simulink model "Bergman_Model_Non_Linear"  (R2026a)
settings: Solver=ode45  StopTime=1440
libraries: mpclib x1
settings Model: Creator=ADMIN
settings SimscapeCC: SimscapeNominalValues="[{\"value\":\"1\",\"unit\":\"A\"},{\"value\":\"1\",\"unit\":\"bar\"},{\"value\":\"1\",\"unit\":\"cm^2\"},{\"value\":\"1\",\"unit\":\"cm^3/s\"},{\"value\":\"1\",\"unit\":\"kJ/kg\"},{\"value\":\"1\",\"unit\":\"kW\"},{\"value\":\"1\",\"unit\":\"l\"},{\"value\":\"1\",\"unit\":\"N\"},{\"value\":\"1\",\"unit\":\"N*m\"},{\"value\":\"1\",\"unit\":\"V\"}]"  SimscapeLogType=none  SimscapeLogDataHistory=5000.0

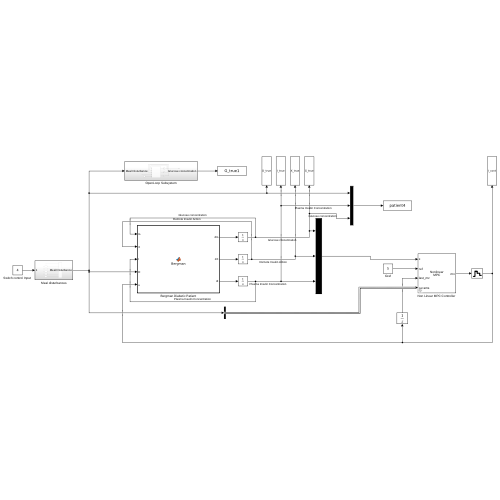
[thumbnail: Simulink's stored preview of the top-level diagram]
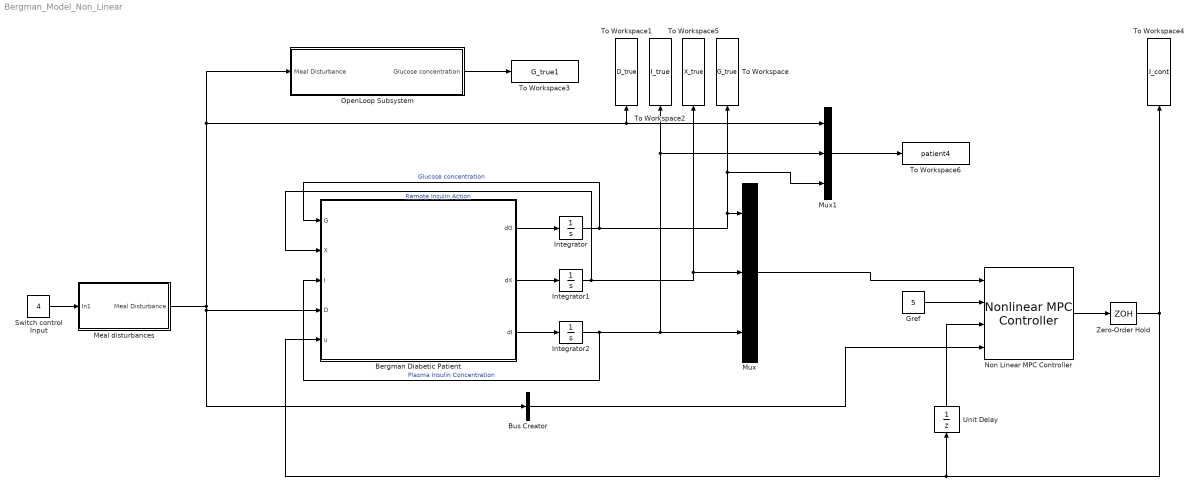
== system Bergman_Model_Non_Linear ==
  Bergman Diabetic Patient : MATLAB Function  TreatAsAtomicUnit=on
  Bus Creator : BusCreator  Inputs=1  OutDataTypeStr=Bus: myParamBus  NonVirtualBus=on
      settings: InheritFromInputs=off
  Gref : Constant  Value=5
  Integrator : Integrator  InitialCondition=5
  Integrator1 : Integrator
  Integrator2 : Integrator
  Meal disturbances : Subsystem
  Mux : Mux  Inputs=3
  Mux1 : Mux  Inputs=3
  "Non Linear MPC Controller " : mpclib/Nonlinear MPC Controller  nlmpcobj=nlobj  md_enabled=off  mvtarget_enabled=off  param_enabled=on  cost_enabled=off  mvseq_enabled=off  stateseq_enabled=off  ovseq_enabled=off  slack_enabled=off  status_enabled=off  ov_min=off  ov_max=off  mv_min=off  mv_max=off  mvrate_min=off  mvrate_max=off  state_min=off  state_max=off  ov_weight=off  mv_weight=off  mvrate_weight=off  ecr_weight=off  nlp_initialize=off  BlockDataType=double  UseObjectTs=on  UseMEX=off
  OpenLoop Subsystem : Subsystem
  "Switch control Input " : Constant  Value=4
  To Workspace : ToWorkspace  VariableName=G_true  SaveFormat=Timeseries  SampleTime=-1
  To Workspace1 : ToWorkspace  VariableName=D_true  SaveFormat=Timeseries  SampleTime=-1
  To Workspace2 : ToWorkspace  VariableName=I_true  SaveFormat=Timeseries  SampleTime=-1
  To Workspace3 : ToWorkspace  VariableName=G_true1  SaveFormat=Timeseries  SampleTime=-1
  To Workspace4 : ToWorkspace  VariableName=I_cont  SaveFormat=Timeseries  SampleTime=-1
  To Workspace5 : ToWorkspace  VariableName=X_true  SaveFormat=Timeseries  SampleTime=-1
  To Workspace6 : ToWorkspace  VariableName=patient4  SaveFormat=Timeseries  SampleTime=-1
  Unit Delay : UnitDelay
  Zero-Order Hold : ZeroOrderHold
  wires:
  Integrator/1 -> Mux1/3, To Workspace/1, Mux/1, Bergman Diabetic Patient/1(G)  "Glucose concentration"
  Integrator1/1 -> Mux/2, To Workspace5/1, Bergman Diabetic Patient/2(X)  "Remote Insulin Action"
  Integrator2/1 -> Mux/3, To Workspace2/1, Mux1/2, Bergman Diabetic Patient/3(I)  "Plasma Insulin Concentration"
  Bergman Diabetic Patient/3(dI) -> Integrator2/1
  Bergman Diabetic Patient/2(dX) -> Integrator1/1
  Bergman Diabetic Patient/1(dG) -> Integrator/1
  Gref/1 -> "Non Linear MPC Controller "/2
  "Non Linear MPC Controller "/1 -> Zero-Order Hold/1
  Unit Delay/1 -> "Non Linear MPC Controller "/3
  Bus Creator/1 -> "Non Linear MPC Controller "/4
  Mux/1 -> "Non Linear MPC Controller "/1
  Zero-Order Hold/1 -> To Workspace4/1, Bergman Diabetic Patient/5(u), Unit Delay/1
  OpenLoop Subsystem/1(Glucose concentration) -> To Workspace3/1
  Meal disturbances/1(Meal Disturbance) -> Bus Creator/1, Bergman Diabetic Patient/4(D), OpenLoop Subsystem/1(Meal Disturbance), To Workspace1/1, Mux1/1
  "Switch control Input "/1 -> Meal disturbances/1(In1)
  Mux1/1 -> To Workspace6/1

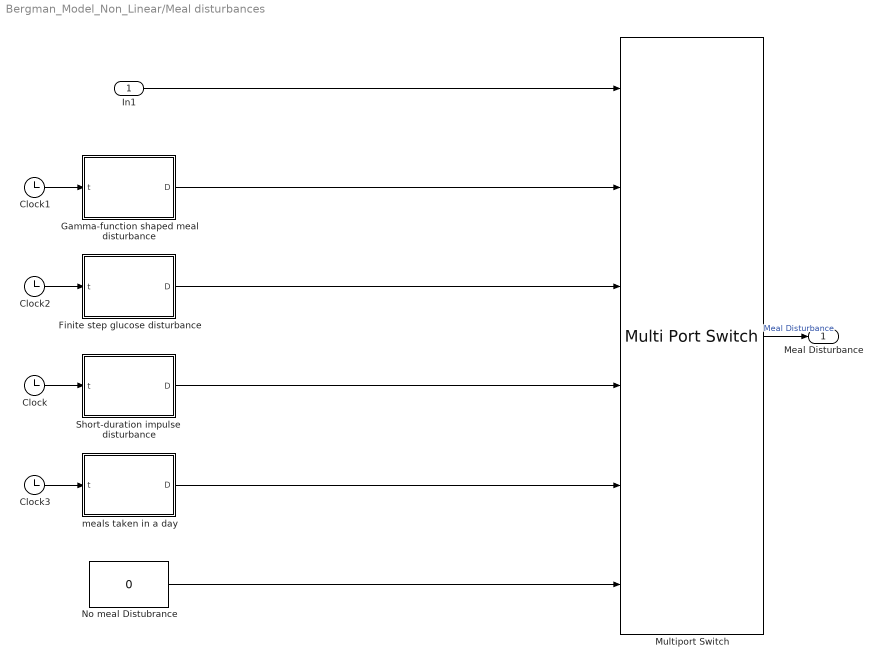
== system Bergman_Model_Non_Linear/Meal disturbances ==
  In1 : Inport
  Clock{,1..3} (4 alike) : Clock
  Finite step glucose disturbance : MATLAB Function  TreatAsAtomicUnit=on
  Gamma-function shaped meal disturbance : MATLAB Function  TreatAsAtomicUnit=on
  Multiport Switch : MultiPortSwitch  Inputs=5  SaturateOnIntegerOverflow=off  InputSameDT=off
  No meal Distubrance : Constant  Value=0
  Short-duration impulse  disturbance : MATLAB Function  TreatAsAtomicUnit=on
  "meals taken in a day " : MATLAB Function  TreatAsAtomicUnit=on
  Meal Disturbance : Outport
  wires:
  Short-duration impulse  disturbance/1(D) -> Multiport Switch/4
  Finite step glucose disturbance/1(D) -> Multiport Switch/3
  "meals taken in a day "/1(D) -> Multiport Switch/5
  Gamma-function shaped meal disturbance/1(D) -> Multiport Switch/2
  Clock/1 -> Short-duration impulse  disturbance/1(t)
  Clock3/1 -> "meals taken in a day "/1(t)
  Clock2/1 -> Finite step glucose disturbance/1(t)
  No meal Distubrance/1 -> Multiport Switch/6
  Clock1/1 -> Gamma-function shaped meal disturbance/1(t)
  In1/1 -> Multiport Switch/1
  Multiport Switch/1 -> Meal Disturbance/1  "Meal Disturbance"

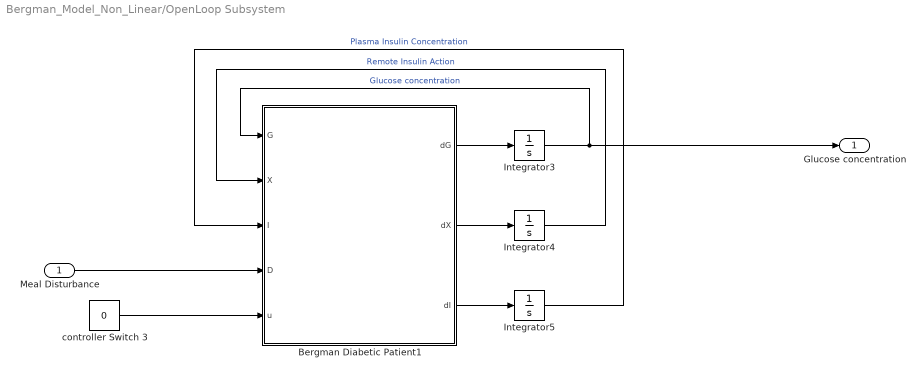
== system Bergman_Model_Non_Linear/OpenLoop Subsystem ==
  Meal Disturbance : Inport
  Bergman Diabetic Patient1 : MATLAB Function  TreatAsAtomicUnit=on
  Integrator3 : Integrator  InitialCondition=5
  Integrator4 : Integrator
  Integrator5 : Integrator
  controller Switch 3 : Constant  Value=0
  Glucose concentration : Outport
  wires:
  controller Switch 3/1 -> Bergman Diabetic Patient1/5(u)
  Integrator5/1 -> Bergman Diabetic Patient1/3(I)  "Plasma Insulin Concentration"
  Integrator4/1 -> Bergman Diabetic Patient1/2(X)  "Remote Insulin Action"
  Bergman Diabetic Patient1/2(dX) -> Integrator4/1
  Bergman Diabetic Patient1/1(dG) -> Integrator3/1
  Bergman Diabetic Patient1/3(dI) -> Integrator5/1
  Integrator3/1 -> Glucose concentration/1, Bergman Diabetic Patient1/1(G)  "Glucose concentration"
  Meal Disturbance/1 -> Bergman Diabetic Patient1/4(D)

== matlab function Bergman_Model_Non_Linear/Meal disturbances/Short-duration impulse  disturbance ==
  data: t input; D output
function D = exponential_meal_disturbance(t)

t_meal = 30;       % Meal occurs at 30 min

k = 0.05;          % 1/min

D0 = 10 * k;        % Total area = 8 mmol/L

if t >= t_meal

    D = D0 * exp(-k*(t - t_meal));

else

    D = 0;

end

end

== matlab function Bergman_Model_Non_Linear/Bergman Diabetic Patient ==
  data: G input; X input; I input; D input; u input; dG output; dX output; dI output
function [dG, dX, dI] = Bergman(G, X, I, D, u)

% Bergman Minimal Model Parameters
p1 = 0.005;
p2 = 0.025;
p3 = 7.00e-5;
n  = 0.0926;

% Basal values
Gb = 5.0;       % mmol/L
Ib = 0;

% State equations
dG    = -p1*(G - Gb) - X*G + D;
dX = -p2*X + p3*max(0, I - Ib);
dI = -n*(I - Ib) + u;

end

== matlab function Bergman_Model_Non_Linear/Meal disturbances/Gamma-function shaped meal disturbance ==
  data: t input; D output
function D = meal_disturbance(t)

t_meal = 30;
tau_D  = 40;

D_max  = 10 / tau_D;   % Gives total area = 10 mmol/L

if t < t_meal

    D = 0.0;

else

    tau = t - t_meal;

    D = D_max * (tau / tau_D) * exp(-tau / tau_D);

end

end

== matlab function Bergman_Model_Non_Linear/Meal disturbances/Finite step glucose disturbance ==
  data: t input; D output
function D = step_disturbance(t)

t_step = 30;          % Meal starts at 30 min
duration = 50;        % Meal lasts 60 min

D_step = 10 / duration;

if t >= t_step && t < (t_step + duration)
    D = D_step;
else
    D = 0.0;
end

end

== matlab function Bergman_Model_Non_Linear/Meal disturbances/meals taken in a day  ==
  data: t input; D output
function D = meals_taken_in_a_day(t)


D = 0.0;


% Breakfast - Gamma-shaped
t_breakfast = 420;      % 07:00 min
tau_B = 40;
A_B = 20;               % Total disturbance area [mmol/L]

Dmax_B = A_B / tau_B;

if t >= t_breakfast

    tau = t - t_breakfast;

    D = Dmax_B * (tau / tau_B) * exp(-tau / tau_B);

end


% Lunch - Step

t_lunch = 720;          % 12:00 min
duration_L = 50;        % Meal duration [min]
A_L = 20;               % Total disturbance area [mmol/L]

Dstep_L = A_L / duration_L;

if t >= t_lunch && t < (t_lunch + duration_L)

    D = D + Dstep_L;

end


% Snack - Exponential

t_snack = 930;          % 15:30 min
A_S = 7;               % Total disturbance area [mmol/L]
k_S = 0.05;             % Decay rate [1/min]

D0_S = A_S * k_S;

if t >= t_snack

    D = D + D0_S * exp(-k_S * (t - t_snack));

end


% Supper - Gamma-shaped

t_supper = 1110;        % 18:30 min
tau_D = 40;
A_D = 30;               % Total disturbance area [mmol/L]

Dmax_D = A_D / tau_D;

if t >= t_supper

    tau = t - t_supper;

    D = D + Dmax_D * (tau / tau_D) * exp(-tau / tau_D);

end

end

== matlab function Bergman_Model_Non_Linear/OpenLoop Subsystem/Bergman Diabetic Patient1 ==
  data: G input; X input; I input; D input; u input; dG output; dX output; dI output
function [dG, dX, dI] = Bergman(G, X, I, D, u)

%bergman minimal model parameters
p1 = 0.005;
p2 = 0.025;
p3 = 5.3e-5;
n  = 0.0926;

%basal values
Gb = 5.0;       % mmol/L
Ib = 0;

%state equations
dG    = -p1*(G - Gb) - X*G + D;
dX = -p2*X + p3*max(0, I - Ib);
dI = -n*(I - Ib) + u;

end
